simulink model "Active_Passive_Balancing"  (R2024b)
settings: Solver=FixedStepDiscrete  StartTime=0.0  StopTime=10  FixedStep=0.02  RelTol=1e-3
settings Model: Creator=mostafa  LastModifiedBy=mostafa
settings OptimizationCC: DefaultParameterBehavior=Inlined  UseDivisionForNetSlopeComputation=on  GainParamInheritBuiltInType=on  UseFloatMulNetSlope=on  InlineInvariantSignals=on  PassReuseOutputArgsAs=Individual arguments  ZeroExternalMemoryAtStartup=off  ZeroInternalMemoryAtStartup=off  NoFixptDivByZeroProtection=on  EfficientFloat2IntCast=on  LifeSpan=1  OptimizeBlockOrder=speed  DifferentSizesBufferReuse=on  EfficientTunableParamExpr=on
settings DebuggingCC: ParameterTunabilityLossMsg=error
settings HardwareCC: ProdLongLongMode=on
settings SFSimCC: MATLABDynamicMemAlloc=off
settings RTWCC: Description=Embedded Coder  SystemTargetFile=ert.tlc  TemplateMakefile=ert_default_tmf  TLCCoverage=on  PortableWordSizes=on  CodeExecutionProfiling=on  CodeStackProfiling=on  SILPILDebugging=on
settings CodeAppCC: ForceParamTrailComments=on  IgnoreCustomStorageClasses=off  OperatorAnnotations=on  SimulinkDataObjDesc=on  SFDataObjDesc=on  CustomSymbolStrGlobalVar=rt$N$M  CustomSymbolStrType=$N$M  CustomSymbolStrFcn=$N$M$F  CustomSymbolStrMacro=$N$M  InsertBlockDesc=on
settings ERTTargetCC: TargetLangStandard=C99 (ISO)  GenerateSampleERTMain=on  IncludeMdlTerminateFcn=off  CombineSignalStateStructs=on  SupportAbsoluteTime=off  SupportComplex=off  SupportNonInlinedSFcns=on  ERTCustomFileTemplate=example_file_process.tlc  ERTFilePackagingFormat=CompactWithDataFile

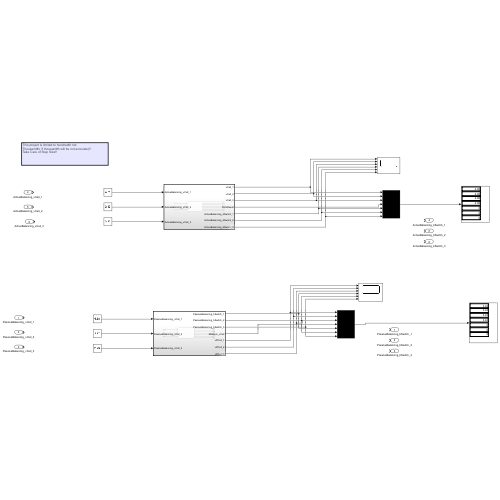
[thumbnail: Simulink's stored preview of the top-level diagram]
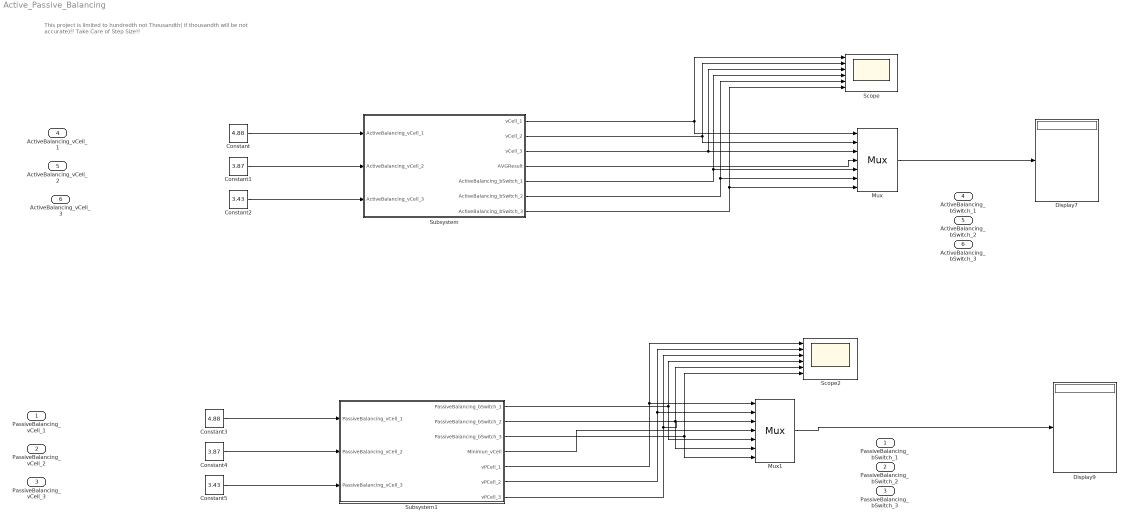
== system Active_Passive_Balancing ==
  note: This project is limited to hundredth not
      | Thousandth( if thousandth will be not accurate)!!
      | Take Care of Step Size!!
  PassiveBalancing_vCell_1 : Inport
  PassiveBalancing_vCell_2 : Inport  Port=2
  PassiveBalancing_vCell_3 : Inport  Port=3
  ActiveBalancing_vCell_1 : Inport  Port=4
  ActiveBalancing_vCell_2 : Inport  Port=5
  ActiveBalancing_vCell_3 : Inport  Port=6
  Constant : Constant  Value=4.88
  Constant1 : Constant  Value=3.87
  Constant2 : Constant  Value=3.43
  Constant3 : Constant  Value=4.88
  Constant4 : Constant  Value=3.87
  Constant5 : Constant  Value=3.43
  Display7 : Display
  Display9 : Display
  Mux : Mux  Inputs=7
  Mux1 : Mux  Inputs=7
  Scope : Scope  NumInputPorts=6
  Scope2 : Scope  NumInputPorts=6
  Subsystem : Subsystem  TreatAsAtomicUnit=on
  Subsystem1 : Subsystem  TreatAsAtomicUnit=on
  PassiveBalancing_bSwitch_1 : Outport
  PassiveBalancing_bSwitch_2 : Outport  Port=2
  PassiveBalancing_bSwitch_3 : Outport  Port=3
  ActiveBalancing_bSwitch_1 : Outport  Port=4
  ActiveBalancing_bSwitch_2 : Outport  Port=5
  ActiveBalancing_bSwitch_3 : Outport  Port=6
  wires:
  Mux/1 -> Display7/1
  Mux1/1 -> Display9/1
  Subsystem/7(ActiveBalancing_bSwitch_3) -> Scope/6, Mux/7
  Subsystem/2(vCell_2) -> Mux/2, Scope/2
  Subsystem/3(vCell_3) -> Mux/3, Scope/3
  Subsystem/5(ActiveBalancing_bSwitch_1) -> Scope/4, Mux/5
  Subsystem/6(ActiveBalancing_bSwitch_2) -> Scope/5, Mux/6
  Subsystem/1(vCell_1) -> Mux/1, Scope/1
  Constant/1 -> Subsystem/1(ActiveBalancing_vCell_1)
  Constant1/1 -> Subsystem/2(ActiveBalancing_vCell_2)
  Constant2/1 -> Subsystem/3(ActiveBalancing_vCell_3)
  Subsystem/4(AVGResult) -> Mux/4
  Subsystem1/1(PassiveBalancing_bSwitch_1) -> Mux1/5, Scope2/4
  Subsystem1/7(vPCell_3) -> Scope2/3, Mux1/3
  Subsystem1/6(vPCell_2) -> Scope2/2, Mux1/2
  Subsystem1/2(PassiveBalancing_bSwitch_2) -> Mux1/6, Scope2/5
  Subsystem1/5(vPCell_1) -> Scope2/1, Mux1/1
  Subsystem1/3(PassiveBalancing_bSwitch_3) -> Mux1/7, Scope2/6
  Constant3/1 -> Subsystem1/1(PassiveBalancing_vCell_1)
  Constant4/1 -> Subsystem1/2(PassiveBalancing_vCell_2)
  Constant5/1 -> Subsystem1/3(PassiveBalancing_vCell_3)
  Subsystem1/4(Minimun_vCell) -> Mux1/4

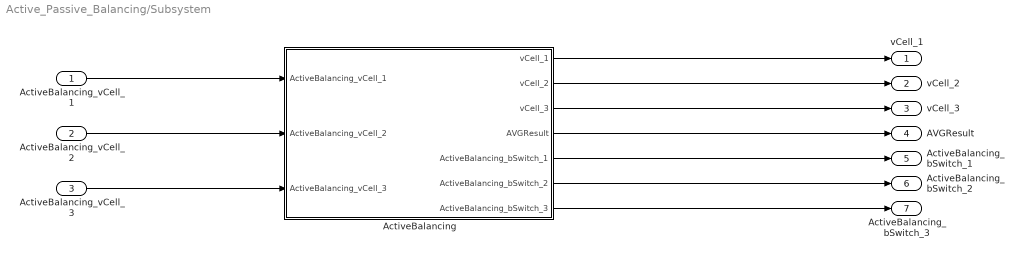
== system Active_Passive_Balancing/Subsystem ==
  ActiveBalancing_vCell_1 : Inport
  ActiveBalancing_vCell_2 : Inport  Port=2
  ActiveBalancing_vCell_3 : Inport  Port=3
  ActiveBalancing : Stateflow chart  TreatAsAtomicUnit=on
  vCell_1 : Outport
  vCell_2 : Outport  Port=2
  vCell_3 : Outport  Port=3
  AVGResult : Outport  Port=4
  ActiveBalancing_bSwitch_1 : Outport  Port=5
  ActiveBalancing_bSwitch_2 : Outport  Port=6
  ActiveBalancing_bSwitch_3 : Outport  Port=7
  wires:
  ActiveBalancing/1(vCell_1) -> vCell_1/1
  ActiveBalancing/7(ActiveBalancing_bSwitch_3) -> ActiveBalancing_bSwitch_3/1
  ActiveBalancing_vCell_1/1 -> ActiveBalancing/1(ActiveBalancing_vCell_1)
  ActiveBalancing/3(vCell_3) -> vCell_3/1
  ActiveBalancing/2(vCell_2) -> vCell_2/1
  ActiveBalancing/4(AVGResult) -> AVGResult/1
  ActiveBalancing/6(ActiveBalancing_bSwitch_2) -> ActiveBalancing_bSwitch_2/1
  ActiveBalancing_vCell_3/1 -> ActiveBalancing/3(ActiveBalancing_vCell_3)
  ActiveBalancing_vCell_2/1 -> ActiveBalancing/2(ActiveBalancing_vCell_2)
  ActiveBalancing/5(ActiveBalancing_bSwitch_1) -> ActiveBalancing_bSwitch_1/1

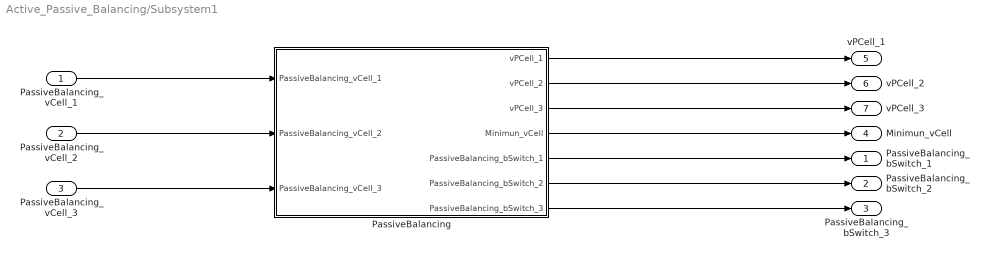
== system Active_Passive_Balancing/Subsystem1 ==
  PassiveBalancing_vCell_1 : Inport
  PassiveBalancing_vCell_2 : Inport  Port=2
  PassiveBalancing_vCell_3 : Inport  Port=3
  PassiveBalancing : Stateflow chart  TreatAsAtomicUnit=on
      settings: PortSchema="{\"entries\":[{\"content\":{\"sides\":[{\"content\":{\"connectorIds\":[\"In1\",\"In2\",\"In3\"]},\"type\":\"ConnectorPlacement.EquallySpacedRectSide\",\"uuid\":\"aba48bfa-ef52-4771-9afa-917bae3ea1e7\"},{\"content\":{\"connectorIds\":[\"Out5\",\"Out6\",\"Out7\",\"Out4\",\"Out1\",\"Out2\",\"Out3\"],\"side\":\"RIGHT\"},\"type\":\"ConnectorPlacement.EquallySpacedRectSide\",\"uuid\":\"97dbb48e-a266-4112-bcf1-fb5106a2ea5e\"},{\"content\":{\"side\":\"TOP\"},\"type\":\"ConnectorPlacement.EquallySpacedRectSide\",\"uuid\":\"3423c9e3-d25c-467f-82d2-d016db26c0c2\"}]},\"type\":\"ConnectorPlacement.EquallySpacedConnector\",\"uuid\":\"6a154df3-3487-427c-a6aa-583e53bde3f3\"}],\"packageUris\":[\"http://schema.mathworks.com/mf0/Connector/R2020b\"],\"version\":\"1.0\"}"
  PassiveBalancing_bSwitch_1 : Outport
  PassiveBalancing_bSwitch_2 : Outport  Port=2
  PassiveBalancing_bSwitch_3 : Outport  Port=3
  Minimun_vCell : Outport  Port=4
  vPCell_1 : Outport  Port=5
  vPCell_2 : Outport  Port=6
  vPCell_3 : Outport  Port=7
  wires:
  PassiveBalancing/5(vPCell_1) -> vPCell_1/1
  PassiveBalancing/4(Minimun_vCell) -> Minimun_vCell/1
  PassiveBalancing/3(PassiveBalancing_bSwitch_3) -> PassiveBalancing_bSwitch_3/1
  PassiveBalancing/6(vPCell_2) -> vPCell_2/1
  PassiveBalancing/7(vPCell_3) -> vPCell_3/1
  PassiveBalancing_vCell_1/1 -> PassiveBalancing/1(PassiveBalancing_vCell_1)
  PassiveBalancing_vCell_3/1 -> PassiveBalancing/3(PassiveBalancing_vCell_3)
  PassiveBalancing/1(PassiveBalancing_bSwitch_1) -> PassiveBalancing_bSwitch_1/1
  PassiveBalancing/2(PassiveBalancing_bSwitch_2) -> PassiveBalancing_bSwitch_2/1
  PassiveBalancing_vCell_2/1 -> PassiveBalancing/2(PassiveBalancing_vCell_2)

== stateflow chart Active_Passive_Balancing/Subsystem1/PassiveBalancing ==
  state SetOutputs [parallel]
    en:
    vPCell_1=PassiveBalancing_vCell_1;
    vPCell_2=PassiveBalancing_vCell_2;
    vPCell_3=PassiveBalancing_vCell_3;
    settings: executionOrder=2
  state Min=Min_Cell(Cell_1,Cell_2,Cell_3) [function]
    (default) -> (junction 546)
    (junction 546) -> (junction 548) [order 1] : [Cell_1<Cell_2&&Cell_1<Cell_3]
    (junction 546) -> (junction 552) [order 2]
    (junction 548) -> (junction 550) : {Min=Cell_1}
    (junction 552) -> (junction 554) [order 1] : [Cell_2<vPCell_1&&Cell_2<Cell_3]
    (junction 552) -> (junction 556) [order 2]
    (junction 554) -> (junction 560) : {Min=Cell_2}
    (junction 556) -> (junction 558) [order 1] : [Cell_3<vPCell_1&&Cell_3<Cell_2]
    (junction 556) -> (junction 565) [order 2]
    (junction 558) -> (junction 562) : {Min=Cell_3}
    (junction 562) -> (junction 565)
    (junction 560) -> (junction 562)
    (junction 550) -> (junction 560)
    (junction 565) -> (junction 570)
  state Cell1 [parallel]
    settings: executionOrder=1
    state CheckingCell1
      (default) -> (junction 247) : {Minimun_vCell=Min_Cell(PassiveBalancing_vCell_1,PassiveBalancing_vCell_2,PassiveBalancing_vCell_3)}
      (junction 247) -> (junction 258) [order 1] : [abs(vPCell_1 - Minimun_vCell) < 0.01]
      (junction 247) -> (junction 249) [order 2] : {PassiveBalancing_bSwitch_1=0}
      (junction 258) -> (junction 250) : {PassiveBalancing_bSwitch_1=1}
      (junction 250) -> (junction 249)
      (junction 249) -> (junction 248)
    state Balancing_Activation_Cell1
      (default) -> (junction 262)
      Balancing_Activation_Cell1 -> (junction 262) [order 1]
      (junction 262) -> (junction 282) [order 1] : [abs(vPCell_1 - Minimun_vCell) <= 0.001]
      (junction 262) -> (junction 276) [order 2]
      (junction 282) -> (junction 279) : {PassiveBalancing_bSwitch_1=0}
      (junction 276) -> (junction 278) [order 1] : [vPCell_1<Minimun_vCell]
      (junction 276) -> (junction 277) [order 2]
      (junction 278) -> (junction 283) : {vPCell_1=vPCell_1+0.01}
      (junction 277) -> (junction 285) [order 1] : [vPCell_1>Minimun_vCell]
      (junction 277) -> (junction 280) [order 2]
      (junction 285) -> (junction 281) : {vPCell_1=vPCell_1-0.01}
      (junction 281) -> (junction 280)
      (junction 283) -> (junction 281)
      (junction 279) -> (junction 283)
      (junction 280) -> (junction 400)
    (default) -> CheckingCell1
    CheckingCell1 -> Balancing_Activation_Cell1 : [PassiveBalancing_bSwitch_1==1]
    Balancing_Activation_Cell1 -> CheckingCell1 [order 1] : [PassiveBalancing_bSwitch_1==0]
  state Cell2 [parallel]
    settings: executionOrder=3
    state Balancing_Activation_Cell2
      (default) -> (junction 454)
      Balancing_Activation_Cell2 -> (junction 454) [order 1]
      (junction 454) -> (junction 446) [order 1] : [abs(vPCell_2 - Minimun_vCell) <= 0.001]
      (junction 454) -> (junction 449) [order 2]
      (junction 446) -> (junction 469) : {PassiveBalancing_bSwitch_2=0}
      (junction 449) -> (junction 447) [order 1] : [vPCell_2<Minimun_vCell]
      (junction 449) -> (junction 453) [order 2]
      (junction 447) -> (junction 473) : {vPCell_2=vPCell_2+0.01}
      (junction 453) -> (junction 455) [order 1] : [vPCell_2>Minimun_vCell]
      (junction 453) -> (junction 450) [order 2]
      (junction 455) -> (junction 451) : {vPCell_2=vPCell_2-0.01}
      (junction 451) -> (junction 450)
      (junction 473) -> (junction 451)
      (junction 469) -> (junction 473)
      (junction 450) -> (junction 477)
    state CheckingCell2
      (default) -> (junction 481) : {Minimun_vCell=Min_Cell(PassiveBalancing_vCell_1,PassiveBalancing_vCell_2,PassiveBalancing_vCell_3)}
      (junction 481) -> (junction 468) [order 1] : [abs(vPCell_2 - Minimun_vCell) > 0.1]
      (junction 481) -> (junction 460) [order 2] : {PassiveBalancing_bSwitch_2=0}
      (junction 468) -> (junction 459) : {PassiveBalancing_bSwitch_2=1}
      (junction 459) -> (junction 460)
      (junction 460) -> (junction 467)
    (default) -> CheckingCell2
    CheckingCell2 -> Balancing_Activation_Cell2 : [PassiveBalancing_bSwitch_2==1]
    Balancing_Activation_Cell2 -> CheckingCell2 [order 1] : [PassiveBalancing_bSwitch_2==0]
  state Cell3 [parallel]
    settings: executionOrder=4
    state Balancing_Activation_Cell3
      (default) -> (junction 499)
      Balancing_Activation_Cell3 -> (junction 499) [order 1]
      (junction 499) -> (junction 491) [order 1] : [abs(vPCell_3 - Minimun_vCell) <= 0.001]
      (junction 499) -> (junction 494) [order 2]
      (junction 491) -> (junction 514) : {PassiveBalancing_bSwitch_3=0}
      (junction 494) -> (junction 492) [order 1] : [vPCell_3<Minimun_vCell]
      (junction 494) -> (junction 498) [order 2]
      (junction 492) -> (junction 518) : {vPCell_3=vPCell_3+0.01}
      (junction 498) -> (junction 500) [order 1] : [vPCell_3>Minimun_vCell]
      (junction 498) -> (junction 495) [order 2]
      (junction 500) -> (junction 496) : {vPCell_3=vPCell_3-0.01}
      (junction 496) -> (junction 495)
      (junction 518) -> (junction 496)
      (junction 514) -> (junction 518)
      (junction 495) -> (junction 522)
    state CheckingCell3
      (default) -> (junction 526) : {Minimun_vCell=Min_Cell(PassiveBalancing_vCell_1,PassiveBalancing_vCell_2,PassiveBalancing_vCell_3)}
      (junction 526) -> (junction 513) [order 1] : [abs(vPCell_3 - Minimun_vCell) > 0.1]
      (junction 526) -> (junction 505) [order 2] : {PassiveBalancing_bSwitch_3=0}
      (junction 513) -> (junction 504) : {PassiveBalancing_bSwitch_3=1}
      (junction 504) -> (junction 505)
      (junction 505) -> (junction 512)
    (default) -> CheckingCell3
    CheckingCell3 -> Balancing_Activation_Cell3 : [PassiveBalancing_bSwitch_3==1]
    Balancing_Activation_Cell3 -> CheckingCell3 [order 1] : [PassiveBalancing_bSwitch_3==0]
  data: Cell_1 function_input double; Cell_2 function_input double; Cell_3 function_input double; Min function_output double; PassiveBalancing_vCell_1 input; PassiveBalancing_vCell_2 input; PassiveBalancing_vCell_3 input; PassiveBalancing_bSwitch_1 output double; PassiveBalancing_bSwitch_2 output double; PassiveBalancing_bSwitch_3 output double; Minimun_vCell output double; vPCell_1 output double; vPCell_2 output double; vPCell_3 output double; Min_Cell local double

== stateflow chart Active_Passive_Balancing/Subsystem/ActiveBalancing ==
  state Avg=GetAvg(Cell1,Cell2,Cell3) [function]
    (default) -> (junction 19) : {Avg=(Cell1+Cell2+Cell3)/3}
  state SetOutputs [parallel]
    en:
    vCell_1=ActiveBalancing_vCell_1;
    vCell_2=ActiveBalancing_vCell_2;
    vCell_3=ActiveBalancing_vCell_3;
    settings: executionOrder=4
  state Cell1 [parallel]
    settings: executionOrder=1
    state Balancing_Activation_Cell1
      (default) -> (junction 262)
      Balancing_Activation_Cell1 -> (junction 262) [order 1]
      (junction 262) -> (junction 282) [order 1] : [abs(vCell_1 - AVGResult) <= 0.001]
      (junction 262) -> (junction 276) [order 2]
      (junction 282) -> (junction 279) : {ActiveBalancing_bSwitch_1=0}
      (junction 276) -> (junction 278) [order 1] : [vCell_1<AVGResult]
      (junction 276) -> (junction 277) [order 2]
      (junction 278) -> (junction 283) : {vCell_1=vCell_1+0.01}
      (junction 277) -> (junction 285) [order 1] : [vCell_1>AVGResult]
      (junction 277) -> (junction 280) [order 2]
      (junction 285) -> (junction 281) : {vCell_1=vCell_1-0.01}
      (junction 281) -> (junction 280)
      (junction 283) -> (junction 281)
      (junction 279) -> (junction 283)
      (junction 280) -> (junction 400)
    state CheckingCell1
      (default) -> (junction 247) : {AVGResult=GetAvg(ActiveBalancing_vCell_1,ActiveBalancing_vCell_2,ActiveBalancing_vCell_3)}
      (junction 247) -> (junction 258) [order 1] : [abs(vCell_1 - AVGResult) > 0.1]
      (junction 247) -> (junction 249) [order 2] : {ActiveBalancing_bSwitch_1=0}
      (junction 258) -> (junction 250) : {ActiveBalancing_bSwitch_1=1}
      (junction 250) -> (junction 249)
      (junction 249) -> (junction 248)
    (default) -> CheckingCell1
    CheckingCell1 -> Balancing_Activation_Cell1 : [ActiveBalancing_bSwitch_1==1]
    Balancing_Activation_Cell1 -> CheckingCell1 [order 1] : [ActiveBalancing_bSwitch_1==0]
  state Cell3 [parallel]
    settings: executionOrder=3
    state Balancing_Activation_Cell3
      (default) -> (junction 368)
      Balancing_Activation_Cell3 -> (junction 368) [order 1]
      (junction 368) -> (junction 402) [order 1] : [abs(vCell_3 - AVGResult) <=0.01]
      (junction 368) -> (junction 371) [order 2]
      (junction 402) -> (junction 359) : {ActiveBalancing_bSwitch_3=0}
      (junction 371) -> (junction 360) [order 1] : [vCell_3<AVGResult]
      (junction 371) -> (junction 356) [order 2]
      (junction 360) -> (junction 375) : {vCell_3=vCell_3+0.01}
      (junction 356) -> (junction 411) [order 1] : [vCell_3>AVGResult]
      (junction 356) -> (junction 357) [order 2]
      (junction 411) -> (junction 363) : {vCell_3=vCell_3-0.01}
      (junction 363) -> (junction 357)
      (junction 375) -> (junction 363)
      (junction 359) -> (junction 375)
      (junction 357) -> (junction 374)
    state CheckingCell3
      (default) -> (junction 337) : {AVGResult=GetAvg(ActiveBalancing_vCell_1,ActiveBalancing_vCell_2,ActiveBalancing_vCell_3)}
      (junction 337) -> (junction 358) [order 1] : [abs(vCell_3 - AVGResult) > 0.1]
      (junction 337) -> (junction 372) [order 2] : {ActiveBalancing_bSwitch_3=0}
      (junction 358) -> (junction 346) : {ActiveBalancing_bSwitch_3=1}
      (junction 346) -> (junction 372)
      (junction 372) -> (junction 338)
    (default) -> CheckingCell3
    CheckingCell3 -> Balancing_Activation_Cell3 : [ActiveBalancing_bSwitch_3==1]
    Balancing_Activation_Cell3 -> CheckingCell3 [order 1] : [ActiveBalancing_bSwitch_3==0]
  state Cell2 [parallel]
    settings: executionOrder=2
    state Balancing_Activation_Cell2
      (default) -> (junction 327)
      Balancing_Activation_Cell2 -> (junction 327) [order 1]
      (junction 327) -> (junction 424) [order 1] : [abs(vCell_2 - AVGResult) <= 0.001]
      (junction 327) -> (junction 330) [order 2]
      (junction 424) -> (junction 318) : {ActiveBalancing_bSwitch_2=0}
      (junction 330) -> (junction 319) [order 1] : [vCell_2<AVGResult]
      (junction 330) -> (junction 315) [order 2]
      (junction 319) -> (junction 334) : {vCell_2=vCell_2+0.01}
      (junction 315) -> (junction 332) [order 2] : [vCell_2>AVGResult]
      (junction 315) -> (junction 316) [order 1]
      (junction 332) -> (junction 322) : {vCell_2=vCell_2-0.01}
      (junction 322) -> (junction 316)
      (junction 334) -> (junction 322)
      (junction 318) -> (junction 334)
      (junction 316) -> (junction 333)
    state CheckingCell2
      (default) -> (junction 296) : {AVGResult=GetAvg(ActiveBalancing_vCell_1,ActiveBalancing_vCell_2,ActiveBalancing_vCell_3)}
      (junction 296) -> (junction 317) [order 1] : [abs(vCell_2 - AVGResult) > 0.01]
      (junction 296) -> (junction 331) [order 2] : {ActiveBalancing_bSwitch_2=0}
      (junction 317) -> (junction 305) : {ActiveBalancing_bSwitch_2=1}
      (junction 305) -> (junction 331)
      (junction 331) -> (junction 297)
    (default) -> CheckingCell2
    CheckingCell2 -> Balancing_Activation_Cell2 : [ActiveBalancing_bSwitch_2==1]
    Balancing_Activation_Cell2 -> CheckingCell2 [order 1] : [ActiveBalancing_bSwitch_2==0]
  data: Cell1 function_input double size=1; Cell2 function_input double size=1; Cell3 function_input double size=1; Avg function_output double size=1; ActiveBalancing_vCell_1 input; ActiveBalancing_vCell_2 input; ActiveBalancing_vCell_3 input; vCell_1 output; vCell_2 output; vCell_3 output; AVGResult output; ActiveBalancing_bSwitch_1 output; ActiveBalancing_bSwitch_2 output; ActiveBalancing_bSwitch_3 output
